simulink model "hw1"  (R2013a)
settings: Solver=ode45  StartTime=0.0  StopTime=10.0  RelTol=1e-3
undefined symbols (not defined in the file): A, B, b, k, r
libraries: simulink x1
settings Model: Creator=admin  LastModifiedBy=admin

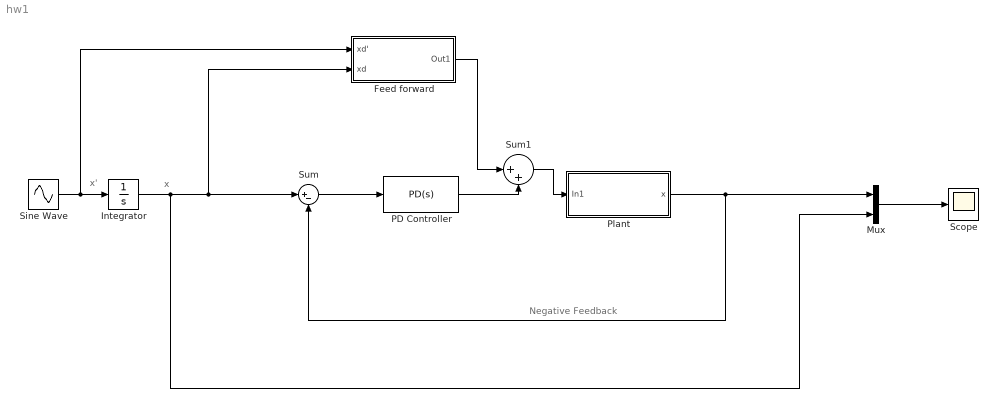
== system hw1 ==
  note: x
  note: x'
  note: Negative Feedback
  Feed forward : Subsystem
  Integrator : Integrator
  Mux : Mux  Inputs=2
  PD Controller : simulink/Continuous/PID Controller  Controller=PD  TimeDomain=Continuous-time  SampleTime=1  IntegratorMethod=Forward Euler  FilterMethod=Forward Euler  Form=Parallel  P=1  I=1  D=0  N=100  InitialConditionSource=internal  InitialConditionForIntegrator=0  InitialConditionForFilter=0  ExternalReset=none  LimitOutput=off  UpperSaturationLimit=inf  LowerSaturationLimit=-inf  LinearizeAsGain=on  AntiWindupMode=none  Kb=1  TrackingMode=off  Kt=1  PParamMin=[]  PParamMax=[]  IParamMin=[]  IParamMax=[]  DParamMin=[]  DParamMax=[]  NParamMin=[]  NParamMax=[]  KbParamMin=[]  KbParamMax=[]  KtParamMin=[]  KtParamMax=[]  POutMin=[]  POutMax=[]  IOutMin=[]  IOutMax=[]  DOutMin=[]  DOutMax=[]  NOutMin=[]  NOutMax=[]  KbOutMin=[]  KbOutMax=[]  KtOutMin=[]  KtOutMax=[]  IntegratorOutMin=[]  IntegratorOutMax=[]  FilterOutMin=[]  FilterOutMax=[]  SumOutMin=[]  SumOutMax=[]  SumI1OutMin=[]  SumI1OutMax=[]  SumI2OutMin=[]  SumI2OutMax=[]  SumI3OutMin=[]  SumI3OutMax=[]  SumDOutMin=[]  SumDOutMax=[]  SaturationOutMin=[]  SaturationOutMax=[]  IntegratorContinuousStateAttributes=''  IntegratorStateMustResolveToSignalObject=off  IntegratorRTWStateStorageClass=Auto  FilterContinuousStateAttributes=''  FilterStateMustResolveToSignalObject=off  FilterRTWStateStorageClass=Auto
  Plant : Subsystem
  Scope : Scope
  Sine Wave : Sin  SampleTime=0
  Sum : Sum  Inputs=|+-
  Sum1 : Sum  Inputs=|++
  wires:
  Mux/1 -> Scope/1
  Sum/1 -> PD Controller/1
  Plant/1(x) -> Mux/1, Sum/2
  Sum1/1 -> Plant/1(In1)
  Feed forward/1(Out1) -> Sum1/1
  Sine Wave/1 -> Feed forward/1(xd'), Integrator/1
  Integrator/1 -> Feed forward/2(xd), Sum/1, Mux/2
  PD Controller/1 -> Sum1/2

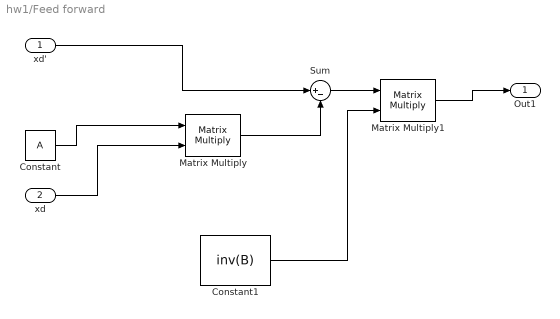
== system hw1/Feed forward ==
  xd' : Inport
  xd : Inport  Port=2
  Constant : Constant  Value=A
  Constant1 : Constant  Value=inv(B)
  Matrix Multiply : Product  Multiplication=Matrix(*)
  Matrix Multiply1 : Product  Multiplication=Matrix(*)
  Sum : Sum  Inputs=|+-
  Out1 : Outport
  wires:
  xd/1 -> Matrix Multiply/2
  Constant/1 -> Matrix Multiply/1
  Matrix Multiply/1 -> Sum/2
  xd'/1 -> Sum/1
  Sum/1 -> Matrix Multiply1/1
  Constant1/1 -> Matrix Multiply1/2
  Matrix Multiply1/1 -> Out1/1

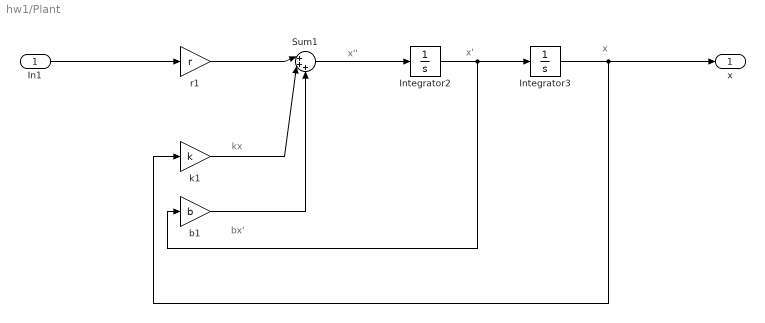
== system hw1/Plant ==
  note: kx
  note: x
  note: x'
  note: x''
  note: bx'
  In1 : Inport
  Integrator2 : Integrator
  Integrator3 : Integrator
  Sum1 : Sum  Inputs=|+++
  b1 : Gain  Gain=b
  k1 : Gain  Gain=k
  r1 : Gain  Gain=r
  x : Outport
  wires:
  k1/1 -> Sum1/2
  r1/1 -> Sum1/1
  b1/1 -> Sum1/3
  Sum1/1 -> Integrator2/1
  Integrator2/1 -> Integrator3/1, b1/1
  Integrator3/1 -> x/1, k1/1
  In1/1 -> r1/1
